simulink model "IPS3_TV_ON_OFF"  (R2019a)
settings: Solver=VariableStepAuto  StartTime=0.0  StopTime=10.0  RelTol=1e-3
settings Model: Creator=Rahulw  LastModifiedBy=Rahulw

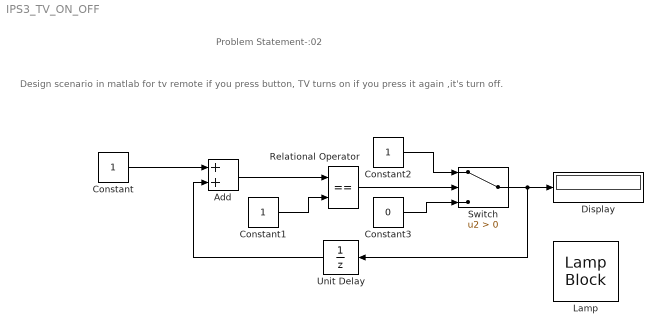
== system IPS3_TV_ON_OFF ==
  note: Design scenario in matlab for tv remote if you press button, TV turns on if you press it again ,it's turn off.
  note: Problem Statement-:02
  Add : Sum
  Constant : Constant
  Constant1 : Constant
  Constant2 : Constant
  Constant3 : Constant  Value=0
  Display : Display
  Lamp : LampBlock
  Relational Operator : RelationalOperator  Operator===  OutDataTypeStr=boolean  RndMeth=Simplest
  Switch : Switch  Criteria=u2 > Threshold
  Unit Delay : UnitDelay  SampleTime=-1  HasFrameUpgradeWarning=on
  wires:
  Constant/1 -> Add/1
  Add/1 -> Relational Operator/1
  Constant1/1 -> Relational Operator/2
  Relational Operator/1 -> Switch/2
  Constant2/1 -> Switch/1
  Constant3/1 -> Switch/3
  Switch/1 -> Unit Delay/1, Display/1
  Unit Delay/1 -> Add/2
